simulink model "Bebop2_sim_only_vis_faster_real_cubic_working_backup"  (R2018a)
settings: Solver=VariableStepAuto  StartTime=0.0  StopTime=25  FixedStep=.04  MaxStep=1.00  MinStep=0.005  RelTol=1e-6  AbsTol=1e-6
values from neighbouring files (symbols this model uses):
  flightplan = [dist,0,height,deg2rad(090) ... (first row only)    [compare_cubic_spline_1.m]    (also in initialize_race_realtime.m; initialize_race_realtime_backup_cubic.m; plot_sim.m = [ 4.348, -0.278, height, deg2rad(  0); test_b_spline.m)
  FOV = 1.05    [initialize_race_realtime.m]    (also in initialize_race_realtime_backup_cubic.m)
  g = 9.81    [initialize_race_no_realtime.m]    (also in initialize_race_realtime.m; initialize_race_realtime_backup_cubic.m; moving_average_rls_own.m = P(i-1)*meas*(lambda+meas*P(i-1)*meas)^-1)
  gate_size = 1.4    [initialize_race_realtime.m]    (also in initialize_race_realtime_backup_cubic.m)
  gates = sim_gates(:,:,1)    [eval_sim.m]    (also in initialize_race_realtime.m = [dist,0,height,deg2rad(110); initialize_race_realtime_backup_cubic.m = [dist,0,height,deg2rad(110); plot_sim.m)
  I = [1 0 0 ... (first row only)    [Bebop_sim_init.m]    (also in initialize_race_no_realtime.m; initialize_race_realtime.m; initialize_race_realtime_backup_cubic.m; moving_averge_rls_download.m = ones(1,N))
  init_std_dev = [1.0*ones(1,3),deg2rad(30)]    [initialize_race_realtime.m]    (also in initialize_race_realtime_backup_cubic.m)
  Initial_ori = [0 0 pi/4]    [initialize_race_no_realtime.m]    (also in initialize_race_realtime.m; initialize_race_realtime_backup_cubic.m)
  Initial_pos = [0 0 1]    [Bebop_sim_init.m]    (also in initialize_race_no_realtime.m = [0 -3 2]; initialize_race_realtime.m = [0 -3 2]; initialize_race_realtime_backup_cubic.m = [0 -3 2])
  Initial_vel_e = max_vel*[1,0,0]    [initialize_race_realtime.m]    (also in initialize_race_realtime_backup_cubic.m)
  m = 0.68    [calc_plot_spline.m]    (also in calc_spline.m; compare_cubic_spline_1.m = vpasolve(e,r); compare_cubic_spline_2.m = r/3*(-sin(dp)+sqrt(sin(dp)^2-6*cos(dp)+6)); initialize_race_no_realtime.m = 2)
  max_rot_Z = (90)*pi/180    (= 1.57079632679)    [Bebop_sim_init.m]    (also in initialize_race_no_realtime.m = 1.0471975512; initialize_race_realtime.m; initialize_race_realtime_backup_cubic.m; run_batch1.m = list_agility(idx_agility)*max_rot_Z)
  max_theta_X = (40)*pi/180    (= 0.698131700798)    [Bebop_sim_init.m]    (also in initialize_race_no_realtime.m = 0.13962634016; initialize_race_realtime.m = 1.308996939; initialize_race_realtime_backup_cubic.m = 1.308996939; run_batch1.m = list_agility(idx_agility)*max_theta_X)
  max_theta_Y = (40)*pi/180    (= 0.698131700798)    [Bebop_sim_init.m]    (also in initialize_race_no_realtime.m = 0.13962634016; initialize_race_realtime.m = 1.308996939; initialize_race_realtime_backup_cubic.m = 1.308996939; run_batch1.m = list_agility(idx_agility)*max_theta_Y)
  max_v_Z = .5    (= 0.5)    [Bebop_sim_init.m]    (also in initialize_race_no_realtime.m = 1; initialize_race_realtime.m = 3; initialize_race_realtime_backup_cubic.m = 3; run_batch1.m = list_agility(idx_agility)*max_v_Z)
  max_vel = 1.5    [initialize_race_realtime.m]    (also in initialize_race_realtime_backup_cubic.m; run_batch1.m = list_speed(idx_speed); run_batch2.m = list_speed(idx_speed); run_batch3.m = list_speed(idx_speed))
undefined symbols (not defined in the file or in its folder): fspecial, gray, Rec, SDTV
libraries: simulink x11, sharedtransform x11, visiontextngfix x4, visiontransforms x3, aerolibactuator x2, aerolibutil x2, vrlib x2, visionanalysis x2, visionconversions x2, shared6dof x1, visionstatistics x1, visionsinks x1
(part 2 of 4)

== system Bebop2_sim_only_vis_faster_real_cubic_working_backup/Vision System/Harris Corners ==
  Threshold : Inport
  Corner Detection : visionanalysis/Corner Detection  method=Harris corner detection (Harris & Stephens)  factor=0.01  filter=fspecial('gaussian', [1 9], 3)  thrInten=0.1  thrAngle=157.5  output=Obsolete9b  outputInUse=Corner location  maxNum=5  thrMetric=0.01  neighborSize=[25 25]  isOutVarDim=on  accumMode=Binary point scaling  accumWordLength=32  accumFracLength=0  prodOutputMode=Binary point scaling  prodOutputWordLength=32  prodOutputFracLength=0  memoryMode=Binary point scaling  memoryWordLength=32  memoryFracLength=0  firstCoeffMode=Specify word length  firstCoeffWordLength=16  firstCoeffFracLength=17  roundingMode=Floor  overflowMode=off
      settings: SourceProductName=Computer Vision System Toolbox  SourceProductBaseCode=VP
  Gaussian Pyramid : visiontransforms/Gaussian Pyramid  Commented=on  operation=Expand  level=1  source=Specify via dialog  a=0.375  coef=fspecial('gaussian', [1 9], 3)  hiddenCoef=fspecial('gaussian', [1 9], 3)  firstCoeffMode=Specify word length  firstCoeffWordLength=16  firstCoeffFracLength=17  outputMode=Binary point scaling  outputWordLength=32  outputFracLength=10  prodOutputMode=Binary point scaling  prodOutputWordLength=32  prodOutputFracLength=10  roundingMode=Floor  overflowMode=off
      settings: SourceProductName=Computer Vision System Toolbox  SourceProductBaseCode=VP
  Video Viewer2 : VideoViewer  Commented=on  colormapValue=gray(256)  FigPos=[76 898 768 763]
  Corners : Outport
  wires:
  Threshold/1 -> Gaussian Pyramid/1, Corner Detection/1
  Gaussian Pyramid/1 -> Video Viewer2/1
  Corner Detection/1 -> Corners/1

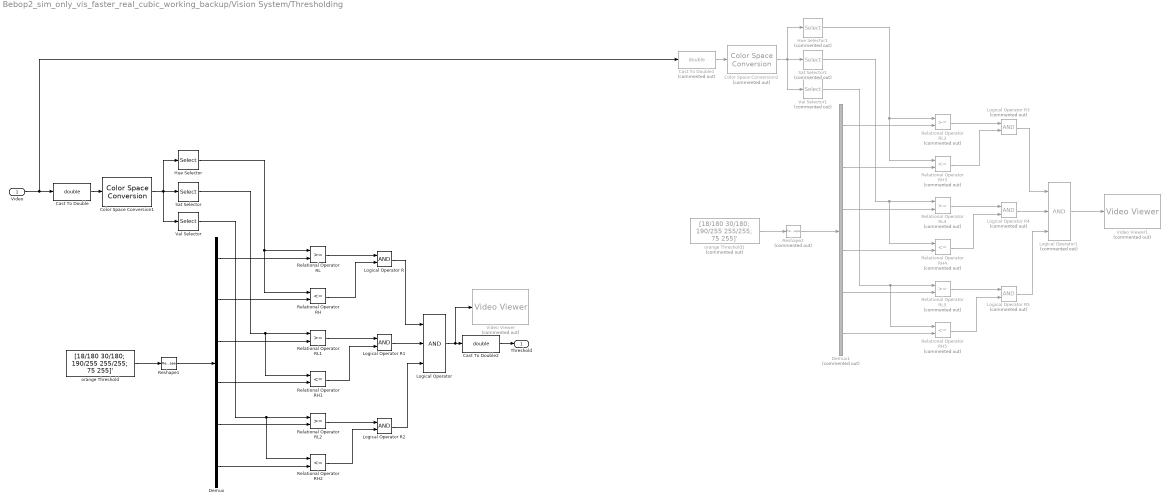
== system Bebop2_sim_only_vis_faster_real_cubic_working_backup/Vision System/Thresholding ==
  "Video " : Inport
  Cast To Double : DataTypeConversion  OutDataTypeStr=double
  Cast To Double1 : DataTypeConversion  Commented=on  OutDataTypeStr=double
  Cast To Double2 : DataTypeConversion  OutDataTypeStr=double
  Color Space Conversion1 : visionconversions/Color Space  Conversion  conversion=Obsolete  conversionActive=R'G'B' to HSV  wp_str=D65  rec=Rec. 601 (SDTV)  sys=1125/60/2:1  imagePorts=One multidimensional signal
      settings: SourceProductName=Computer Vision System Toolbox
  Color Space Conversion2 : visionconversions/Color Space  Conversion  Commented=on  conversion=Obsolete  conversionActive=R'G'B' to HSV  wp_str=D65  rec=Rec. 601 (SDTV)  sys=1125/60/2:1  imagePorts=One multidimensional signal
      settings: SourceProductName=Computer Vision System Toolbox
  Demux : Demux  Outputs=6
  Demux1 : Demux  Commented=on  Outputs=6
  Hue Selector : Selector  NumberOfDimensions=3  IndexMode=Zero-based  InputPortWidth=3  IndexOptions=Select all,Select all,Index vector (dialog)  Indices=[1 3],1,0  OutputSizes=1,1,1
  Hue Selector1 : Selector  Commented=on  NumberOfDimensions=3  InputPortWidth=3  IndexOptions=Select all,Select all,Index vector (dialog)  Indices=[1 3],1,1  OutputSizes=1,1,1
  Logical Operator : Logic  Inputs=3  AllPortsSameDT=off  OutDataTypeStr=boolean
  Logical Operator R : Logic  AllPortsSameDT=off  OutDataTypeStr=boolean
  Logical Operator R1 : Logic  AllPortsSameDT=off  OutDataTypeStr=boolean
  Logical Operator R2 : Logic  AllPortsSameDT=off  OutDataTypeStr=boolean
  Logical Operator R3 : Logic  Commented=on  AllPortsSameDT=off  OutDataTypeStr=boolean
  Logical Operator R4 : Logic  Commented=on  AllPortsSameDT=off  OutDataTypeStr=boolean
  Logical Operator R5 : Logic  Commented=on  AllPortsSameDT=off  OutDataTypeStr=boolean
  Logical Operator1 : Logic  Commented=on  Inputs=3  AllPortsSameDT=off  OutDataTypeStr=boolean
  Relational Operator RH : RelationalOperator  Operator=<=  OutDataTypeStr=boolean  RndMeth=Nearest
  Relational Operator RH1 : RelationalOperator  Operator=<=  OutDataTypeStr=boolean  RndMeth=Nearest
  Relational Operator RH2 : RelationalOperator  Operator=<=  OutDataTypeStr=boolean  RndMeth=Nearest
  Relational Operator RH3 : RelationalOperator  Commented=on  Operator=<=  OutDataTypeStr=boolean  RndMeth=Nearest
  Relational Operator RH4 : RelationalOperator  Commented=on  Operator=<=  OutDataTypeStr=boolean  RndMeth=Nearest
  Relational Operator RH5 : RelationalOperator  Commented=on  Operator=<=  OutDataTypeStr=boolean  RndMeth=Nearest
  Relational Operator RL : RelationalOperator  OutDataTypeStr=boolean  RndMeth=Nearest
  Relational Operator RL1 : RelationalOperator  OutDataTypeStr=boolean  RndMeth=Nearest
  Relational Operator RL2 : RelationalOperator  OutDataTypeStr=boolean  RndMeth=Nearest
  Relational Operator RL3 : RelationalOperator  Commented=on  OutDataTypeStr=boolean  RndMeth=Nearest
  Relational Operator RL4 : RelationalOperator  Commented=on  OutDataTypeStr=boolean  RndMeth=Nearest
  Relational Operator RL5 : RelationalOperator  Commented=on  OutDataTypeStr=boolean  RndMeth=Nearest
  Reshape1 : Reshape
  Reshape2 : Reshape  Commented=on
  Sat Selector : Selector  NumberOfDimensions=3  IndexMode=Zero-based  InputPortWidth=3  IndexOptions=Select all,Select all,Index vector (dialog)  Indices=[1 3],1,1  OutputSizes=1,1,1
  Sat Selector1 : Selector  Commented=on  NumberOfDimensions=3  InputPortWidth=3  IndexOptions=Select all,Select all,Index vector (dialog)  Indices=[1 3],1,2  OutputSizes=1,1,1
  Val Selector : Selector  NumberOfDimensions=3  IndexMode=Zero-based  InputPortWidth=3  IndexOptions=Select all,Select all,Index vector (dialog)  Indices=[1 3],1,2  OutputSizes=1,1,1
  Val Selector1 : Selector  Commented=on  NumberOfDimensions=3  InputPortWidth=3  IndexOptions=Select all,Select all,Index vector (dialog)  Indices=[1 3],1,3  OutputSizes=1,1,1
  Video Viewer : VideoViewer  Commented=on  colormapValue=gray(256)  FigPos=[833 898 768 793]
  Video Viewer1 : VideoViewer  Commented=on  colormapValue=gray(256)  FigPos=[823 898 778 793]
  orange Threshold : Constant  Value=[18/180 30/180; 190/255 255/255; 75 255]'  OutDataTypeStr=double
  orange Threshold1 : Constant  Commented=on  Value=[18/180 30/180; 190/255 255/255; 75 255]'  OutDataTypeStr=double
  Threshold : Outport
  wires:
  Color Space Conversion1/1 -> Val Selector/1, Sat Selector/1, Hue Selector/1
  Demux/6 -> Relational Operator RH2/2
  Val Selector/1 -> Relational Operator RH2/1, Relational Operator RL2/1
  Demux/3 -> Relational Operator RL1/2
  Relational Operator RL/1 -> Logical Operator R/1
  Demux/2 -> Relational Operator RH/2
  orange Threshold/1 -> Reshape1/1
  Cast To Double/1 -> Color Space Conversion1/1
  Demux/5 -> Relational Operator RL2/2
  Hue Selector/1 -> Relational Operator RH/1, Relational Operator RL/1
  Logical Operator R/1 -> Logical Operator/1
  Relational Operator RH/1 -> Logical Operator R/2
  Demux/1 -> Relational Operator RL/2
  Demux/4 -> Relational Operator RH1/2
  Reshape1/1 -> Demux/1
  Logical Operator R1/1 -> Logical Operator/2
  Relational Operator RH1/1 -> Logical Operator R1/2
  Sat Selector/1 -> Relational Operator RH1/1, Relational Operator RL1/1
  Relational Operator RL1/1 -> Logical Operator R1/1
  Relational Operator RH2/1 -> Logical Operator R2/2
  Relational Operator RL2/1 -> Logical Operator R2/1
  Logical Operator R2/1 -> Logical Operator/3
  Logical Operator/1 -> Video Viewer/1, Cast To Double2/1
  Demux1/5 -> Relational Operator RL5/2
  Relational Operator RH3/1 -> Logical Operator R3/2
  orange Threshold1/1 -> Reshape2/1
  Demux1/1 -> Relational Operator RL3/2
  Relational Operator RH4/1 -> Logical Operator R4/2
  Demux1/4 -> Relational Operator RH4/2
  Relational Operator RH5/1 -> Logical Operator R5/2
  Logical Operator R5/1 -> Logical Operator1/3
  Relational Operator RL4/1 -> Logical Operator R4/1
  Demux1/6 -> Relational Operator RH5/2
  Demux1/2 -> Relational Operator RH3/2
  Reshape2/1 -> Demux1/1
  Logical Operator1/1 -> Video Viewer1/1
  Hue Selector1/1 -> Relational Operator RH3/1, Relational Operator RL3/1
  Color Space Conversion2/1 -> Val Selector1/1, Sat Selector1/1, Hue Selector1/1
  Logical Operator R3/1 -> Logical Operator1/1
  Cast To Double1/1 -> Color Space Conversion2/1
  Demux1/3 -> Relational Operator RL4/2
  Relational Operator RL3/1 -> Logical Operator R3/1
  Val Selector1/1 -> Relational Operator RH5/1, Relational Operator RL5/1
  Relational Operator RL5/1 -> Logical Operator R5/1
  Logical Operator R4/1 -> Logical Operator1/2
  "Video "/1 -> Cast To Double1/1, Cast To Double/1
  Sat Selector1/1 -> Relational Operator RH4/1, Relational Operator RL4/1
  Cast To Double2/1 -> Threshold/1

== system Bebop2_sim_only_vis_faster_real_cubic_working_backup/Vision System/calculate corners ==
  In1 : Inport
  Action Port : ActionPort  PropagateVarSize=During execution  ActionType=then
  calculate corners : MATLAB Function  TreatAsAtomicUnit=on
  Out1 : Outport
  wires:
  In1/1 -> calculate corners/1(corners)
  calculate corners/1(corners_four) -> Out1/1

== system Bebop2_sim_only_vis_faster_real_cubic_working_backup/conv/global2strange drone ==
  note: rotm2axang(m1*m2)
  note: eul2rotm([-pi/2, 0, pi/2])
  note: eul2rotm([euler(3),euler(2),euler(1)])
  euler global : Inport
  Constant : Constant  Value=pi/2
  Constant1 : Constant  Value=0
  Direction Cosine Matrix to Quaternions : sharedtransform/Direction Cosine Matrix  to Quaternions  aMode=0  action=None  tolerance=eps(2)
      settings: SourceProductName=Aerospace Blockset  SourceProductBaseCode=AE
  Gain : Gain  Gain=-1
  Gain2 : Gain  Gain=-1
  Gain3 : Gain  Gain=[-1,-1,-1,1]
  MATLAB Function : MATLAB Function  Commented=on  TreatAsAtomicUnit=on
  MATLAB Function1 : MATLAB Function  TreatAsAtomicUnit=on
  Matrix Multiply : Product  Multiplication=Matrix(*)
  Rotation Angles to Direction Cosine Matrix : sharedtransform/Rotation Angles to Direction Cosine Matrix  rotationOrder=XYZ  aMode=aMode
      settings: SourceProductBaseCode=AE
  Rotation Angles to Direction Cosine Matrix1 : sharedtransform/Rotation Angles to Direction Cosine Matrix  rotationOrder=XYZ  aMode=aMode
      settings: SourceProductBaseCode=AE
  Vector Concatenate : Concatenate  NumInputs=3
  axang strange : Outport
  wires:
  Constant/1 -> Vector Concatenate/3, Gain/1
  Constant1/1 -> Vector Concatenate/2
  Gain/1 -> Vector Concatenate/1
  Rotation Angles to Direction Cosine Matrix/1 -> Matrix Multiply/2
  euler global/1 -> Gain2/1
  Rotation Angles to Direction Cosine Matrix1/1 -> Matrix Multiply/1
  Matrix Multiply/1 -> Direction Cosine Matrix to Quaternions/1
  MATLAB Function1/1(axang) -> Gain3/1
  Vector Concatenate/1 -> Rotation Angles to Direction Cosine Matrix/1
  Gain2/1 -> Rotation Angles to Direction Cosine Matrix1/1
  Direction Cosine Matrix to Quaternions/1 -> MATLAB Function1/1(q)
  Gain3/1 -> axang strange/1

== system Bebop2_sim_only_vis_faster_real_cubic_working_backup/Control/Control algorithm/Create Path Frame ==
  Velocity Vector : Inport
  Invert 3x3 Matrix : aerolibutil/Invert  3x3 Matrix
  Make X Vector : Subsystem
  Make Y Vector : Subsystem
  Make Z Vector : Subsystem
  Matrix Concatenate : Concatenate  NumInputs=3  Mode=Multidimensional array  ConcatenateDimension=2
  Rotation Matrix : Outport
  wires:
  Velocity Vector/1 -> Make Z Vector/1(Velocity Vector), Make X Vector/1(Velocity Vector), Make Y Vector/1(Velocity Vector)
  Make Y Vector/1(Y Vector) -> Matrix Concatenate/2
  Make X Vector/1(X Vector) -> Matrix Concatenate/1
  Make Z Vector/1(Z Vector) -> Matrix Concatenate/3
  Matrix Concatenate/1 -> Invert 3x3 Matrix/1
  Invert 3x3 Matrix/1 -> Rotation Matrix/1

== system Bebop2_sim_only_vis_faster_real_cubic_working_backup/Control/Control algorithm/Hdg Controller R ==
  delta yaw : Inport
  Atan2 : Trigonometry  Operator=atan2
  Cos : Trigonometry  Operator=sincos
  PID Controller 0.075 : simulink/Continuous/PID Controller  Controller=PID  TimeDomain=Continuous-time  SampleTime=-1  IntegratorMethod=Forward Euler  FilterMethod=Forward Euler  Form=Parallel  UseFilter=on  ControllerParametersSource=internal  P=9  I=0  D=.9  N=100  InitialConditionSource=internal  InitialConditionForIntegrator=0  InitialConditionForFilter=0  ExternalReset=none  LimitOutput=off  UpperSaturationLimit=inf  LowerSaturationLimit=-inf  LinearizeAsGain=on  AntiWindupMode=none  Kb=1  TrackingMode=off  Kt=1  PParamMin=[]  PParamMax=[]  IParamMin=[]  IParamMax=[]  DParamMin=[]  DParamMax=[]  NParamMin=[]  NParamMax=[]  KbParamMin=[]  KbParamMax=[]  KtParamMin=[]  KtParamMax=[]  POutMin=[]  POutMax=[]  IOutMin=[]  IOutMax=[]  DOutMin=[]  DOutMax=[]  NOutMin=[]  NOutMax=[]  KbOutMin=[]  KbOutMax=[]  KtOutMin=[]  KtOutMax=[]  IntegratorOutMin=[]  IntegratorOutMax=[]  FilterOutMin=[]  FilterOutMax=[]  SumOutMin=[]  SumOutMax=[]  SumI1OutMin=[]  SumI1OutMax=[]  SumI2OutMin=[]  SumI2OutMax=[]  SumI3OutMin=[]  SumI3OutMax=[]  SumDOutMin=[]  SumDOutMax=[]  SaturationOutMin=[]  SaturationOutMax=[]  IntegratorContinuousStateAttributes=''  IntegratorStateMustResolveToSignalObject=off  IntegratorRTWStateStorageClass=Auto  FilterContinuousStateAttributes=''  FilterStateMustResolveToSignalObject=off  FilterRTWStateStorageClass=Auto  DifferentiatorICPrevScaledInput=0  DifferentiatorOutMin=[]  DifferentiatorOutMax=[]  FilterDiffOutCoefMin=[]  FilterDiffOutCoefMax=[]  SumDenOutMin=[]  SumDenOutMax=[]  SumNumOutMin=[]  SumNumOutMax=[]  ReciprocalOutMin=[]  ReciprocalOutMax=[]  DivideOutMin=[]  DivideOutMax=[]  TunerSelectOption=Transfer Function Based (PID Tuner App)
  PID Controller 0.15 : simulink/Continuous/PID Controller  Controller=PID  TimeDomain=Continuous-time  SampleTime=-1  IntegratorMethod=Forward Euler  FilterMethod=Forward Euler  Form=Parallel  UseFilter=on  ControllerParametersSource=internal  P=4  I=0  D=0  N=100  InitialConditionSource=internal  InitialConditionForIntegrator=0  InitialConditionForFilter=0  ExternalReset=none  LimitOutput=off  UpperSaturationLimit=inf  LowerSaturationLimit=-inf  LinearizeAsGain=on  AntiWindupMode=none  Kb=1  TrackingMode=off  Kt=1  PParamMin=[]  PParamMax=[]  IParamMin=[]  IParamMax=[]  DParamMin=[]  DParamMax=[]  NParamMin=[]  NParamMax=[]  KbParamMin=[]  KbParamMax=[]  KtParamMin=[]  KtParamMax=[]  POutMin=[]  POutMax=[]  IOutMin=[]  IOutMax=[]  DOutMin=[]  DOutMax=[]  NOutMin=[]  NOutMax=[]  KbOutMin=[]  KbOutMax=[]  KtOutMin=[]  KtOutMax=[]  IntegratorOutMin=[]  IntegratorOutMax=[]  FilterOutMin=[]  FilterOutMax=[]  SumOutMin=[]  SumOutMax=[]  SumI1OutMin=[]  SumI1OutMax=[]  SumI2OutMin=[]  SumI2OutMax=[]  SumI3OutMin=[]  SumI3OutMax=[]  SumDOutMin=[]  SumDOutMax=[]  SaturationOutMin=[]  SaturationOutMax=[]  IntegratorContinuousStateAttributes=''  IntegratorStateMustResolveToSignalObject=off  IntegratorRTWStateStorageClass=Auto  FilterContinuousStateAttributes=''  FilterStateMustResolveToSignalObject=off  FilterRTWStateStorageClass=Auto  DifferentiatorICPrevScaledInput=0  DifferentiatorOutMin=[]  DifferentiatorOutMax=[]  FilterDiffOutCoefMin=[]  FilterDiffOutCoefMax=[]  SumDenOutMin=[]  SumDenOutMax=[]  SumNumOutMin=[]  SumNumOutMax=[]  ReciprocalOutMin=[]  ReciprocalOutMax=[]  DivideOutMin=[]  DivideOutMax=[]  TunerSelectOption=Transfer Function Based (PID Tuner App)
  PID Controller 0.15 p : simulink/Continuous/PID Controller  Controller=PID  TimeDomain=Continuous-time  SampleTime=-1  IntegratorMethod=Forward Euler  FilterMethod=Forward Euler  Form=Parallel  UseFilter=on  ControllerParametersSource=internal  P=3  I=0  D=0  N=100  InitialConditionSource=internal  InitialConditionForIntegrator=0  InitialConditionForFilter=0  ExternalReset=none  LimitOutput=off  UpperSaturationLimit=inf  LowerSaturationLimit=-inf  LinearizeAsGain=on  AntiWindupMode=none  Kb=1  TrackingMode=off  Kt=1  PParamMin=[]  PParamMax=[]  IParamMin=[]  IParamMax=[]  DParamMin=[]  DParamMax=[]  NParamMin=[]  NParamMax=[]  KbParamMin=[]  KbParamMax=[]  KtParamMin=[]  KtParamMax=[]  POutMin=[]  POutMax=[]  IOutMin=[]  IOutMax=[]  DOutMin=[]  DOutMax=[]  NOutMin=[]  NOutMax=[]  KbOutMin=[]  KbOutMax=[]  KtOutMin=[]  KtOutMax=[]  IntegratorOutMin=[]  IntegratorOutMax=[]  FilterOutMin=[]  FilterOutMax=[]  SumOutMin=[]  SumOutMax=[]  SumI1OutMin=[]  SumI1OutMax=[]  SumI2OutMin=[]  SumI2OutMax=[]  SumI3OutMin=[]  SumI3OutMax=[]  SumDOutMin=[]  SumDOutMax=[]  SaturationOutMin=[]  SaturationOutMax=[]  IntegratorContinuousStateAttributes=''  IntegratorStateMustResolveToSignalObject=off  IntegratorRTWStateStorageClass=Auto  FilterContinuousStateAttributes=''  FilterStateMustResolveToSignalObject=off  FilterRTWStateStorageClass=Auto  DifferentiatorICPrevScaledInput=0  DifferentiatorOutMin=[]  DifferentiatorOutMax=[]  FilterDiffOutCoefMin=[]  FilterDiffOutCoefMax=[]  SumDenOutMin=[]  SumDenOutMax=[]  SumNumOutMin=[]  SumNumOutMax=[]  ReciprocalOutMin=[]  ReciprocalOutMax=[]  DivideOutMin=[]  DivideOutMax=[]  TunerSelectOption=Transfer Function Based (PID Tuner App)
  yaw rate : Outport
  wires:
  delta yaw/1 -> Cos/1  "delta yaw"
  Cos/1 -> Atan2/1
  PID Controller 0.075/1 -> yaw rate/1  "yaw rate"
  Atan2/1 -> PID Controller 0.075/1  "d yaw"
  Cos/2 -> Atan2/2

== system Bebop2_sim_only_vis_faster_real_cubic_working_backup/Control/Control algorithm/Orientation to 3D yaw rotation ==
  Drone yaw : Inport
  Constant1 : Constant  Value=0
  Rotation Angles to Direction Cosine Matrix : sharedtransform/Rotation Angles to Direction Cosine Matrix  rotationOrder=ZYX  aMode=aMode
      settings: SourceProductBaseCode=AE
  Vector Concatenate : Concatenate  NumInputs=3
  rot matrix : Outport
  wires:
  Constant1/1 -> Vector Concatenate/2, Vector Concatenate/3
  Vector Concatenate/1 -> Rotation Angles to Direction Cosine Matrix/1
  Drone yaw/1 -> Vector Concatenate/1  "yaw"
  Rotation Angles to Direction Cosine Matrix/1 -> rot matrix/1  "rot matrix"

== system Bebop2_sim_only_vis_faster_real_cubic_working_backup/Control/Control algorithm/Vel Controller X,Y1 ==
  note: 0.075
  note: 0.15
  note: 0.075
  delta V traj : Inport
  Demux1 : Demux  Outputs=3
  Gain3 : Gain  Gain=2
  Gain4 : Gain  Gain=8
  Gain5 : Gain  Gain=2.5
  Gain6 : Gain  Gain=.75
  Gain7 : Gain  Gain=3
  Gain8 : Gain  Gain=1.25
  Mux : Mux  Inputs=3
  PID Controller1 : simulink/Continuous/PID Controller  Controller=PID  TimeDomain=Continuous-time  SampleTime=-1  IntegratorMethod=Forward Euler  FilterMethod=Forward Euler  Form=Parallel  UseFilter=on  ControllerParametersSource=internal  P=2  I=0  D=0  N=100  InitialConditionSource=internal  InitialConditionForIntegrator=0  InitialConditionForFilter=0  ExternalReset=none  LimitOutput=off  UpperSaturationLimit=inf  LowerSaturationLimit=-inf  LinearizeAsGain=on  AntiWindupMode=none  Kb=1  TrackingMode=off  Kt=1  PParamMin=[]  PParamMax=[]  IParamMin=[]  IParamMax=[]  DParamMin=[]  DParamMax=[]  NParamMin=[]  NParamMax=[]  KbParamMin=[]  KbParamMax=[]  KtParamMin=[]  KtParamMax=[]  POutMin=[]  POutMax=[]  IOutMin=[]  IOutMax=[]  DOutMin=[]  DOutMax=[]  NOutMin=[]  NOutMax=[]  KbOutMin=[]  KbOutMax=[]  KtOutMin=[]  KtOutMax=[]  IntegratorOutMin=[]  IntegratorOutMax=[]  FilterOutMin=[]  FilterOutMax=[]  SumOutMin=[]  SumOutMax=[]  SumI1OutMin=[]  SumI1OutMax=[]  SumI2OutMin=[]  SumI2OutMax=[]  SumI3OutMin=[]  SumI3OutMax=[]  SumDOutMin=[]  SumDOutMax=[]  SaturationOutMin=[]  SaturationOutMax=[]  IntegratorContinuousStateAttributes=''  IntegratorStateMustResolveToSignalObject=off  IntegratorRTWStateStorageClass=Auto  FilterContinuousStateAttributes=''  FilterStateMustResolveToSignalObject=off  FilterRTWStateStorageClass=Auto  DifferentiatorICPrevScaledInput=0  DifferentiatorOutMin=[]  DifferentiatorOutMax=[]  FilterDiffOutCoefMin=[]  FilterDiffOutCoefMax=[]  SumDenOutMin=[]  SumDenOutMax=[]  SumNumOutMin=[]  SumNumOutMax=[]  ReciprocalOutMin=[]  ReciprocalOutMax=[]  DivideOutMin=[]  DivideOutMax=[]  TunerSelectOption=Transfer Function Based (PID Tuner App)
  PID Controller2 : simulink/Continuous/PID Controller  Controller=PID  TimeDomain=Continuous-time  SampleTime=-1  IntegratorMethod=Forward Euler  FilterMethod=Forward Euler  Form=Parallel  UseFilter=on  ControllerParametersSource=internal  P=6  I=0  D=.9  N=100  InitialConditionSource=internal  InitialConditionForIntegrator=0  InitialConditionForFilter=0  ExternalReset=none  LimitOutput=off  UpperSaturationLimit=inf  LowerSaturationLimit=-inf  LinearizeAsGain=on  AntiWindupMode=none  Kb=1  TrackingMode=off  Kt=1  PParamMin=[]  PParamMax=[]  IParamMin=[]  IParamMax=[]  DParamMin=[]  DParamMax=[]  NParamMin=[]  NParamMax=[]  KbParamMin=[]  KbParamMax=[]  KtParamMin=[]  KtParamMax=[]  POutMin=[]  POutMax=[]  IOutMin=[]  IOutMax=[]  DOutMin=[]  DOutMax=[]  NOutMin=[]  NOutMax=[]  KbOutMin=[]  KbOutMax=[]  KtOutMin=[]  KtOutMax=[]  IntegratorOutMin=[]  IntegratorOutMax=[]  FilterOutMin=[]  FilterOutMax=[]  SumOutMin=[]  SumOutMax=[]  SumI1OutMin=[]  SumI1OutMax=[]  SumI2OutMin=[]  SumI2OutMax=[]  SumI3OutMin=[]  SumI3OutMax=[]  SumDOutMin=[]  SumDOutMax=[]  SaturationOutMin=[]  SaturationOutMax=[]  IntegratorContinuousStateAttributes=''  IntegratorStateMustResolveToSignalObject=off  IntegratorRTWStateStorageClass=Auto  FilterContinuousStateAttributes=''  FilterStateMustResolveToSignalObject=off  FilterRTWStateStorageClass=Auto  DifferentiatorICPrevScaledInput=0  DifferentiatorOutMin=[]  DifferentiatorOutMax=[]  FilterDiffOutCoefMin=[]  FilterDiffOutCoefMax=[]  SumDenOutMin=[]  SumDenOutMax=[]  SumNumOutMin=[]  SumNumOutMax=[]  ReciprocalOutMin=[]  ReciprocalOutMax=[]  DivideOutMin=[]  DivideOutMax=[]  TunerSelectOption=Transfer Function Based (PID Tuner App)
  PID Controller3 : simulink/Continuous/PID Controller  Controller=PID  TimeDomain=Continuous-time  SampleTime=-1  IntegratorMethod=Forward Euler  FilterMethod=Forward Euler  Form=Parallel  UseFilter=on  ControllerParametersSource=internal  P=1  I=0  D=0  N=100  InitialConditionSource=internal  InitialConditionForIntegrator=0  InitialConditionForFilter=0  ExternalReset=none  LimitOutput=off  UpperSaturationLimit=inf  LowerSaturationLimit=-inf  LinearizeAsGain=on  AntiWindupMode=none  Kb=1  TrackingMode=off  Kt=1  PParamMin=[]  PParamMax=[]  IParamMin=[]  IParamMax=[]  DParamMin=[]  DParamMax=[]  NParamMin=[]  NParamMax=[]  KbParamMin=[]  KbParamMax=[]  KtParamMin=[]  KtParamMax=[]  POutMin=[]  POutMax=[]  IOutMin=[]  IOutMax=[]  DOutMin=[]  DOutMax=[]  NOutMin=[]  NOutMax=[]  KbOutMin=[]  KbOutMax=[]  KtOutMin=[]  KtOutMax=[]  IntegratorOutMin=[]  IntegratorOutMax=[]  FilterOutMin=[]  FilterOutMax=[]  SumOutMin=[]  SumOutMax=[]  SumI1OutMin=[]  SumI1OutMax=[]  SumI2OutMin=[]  SumI2OutMax=[]  SumI3OutMin=[]  SumI3OutMax=[]  SumDOutMin=[]  SumDOutMax=[]  SaturationOutMin=[]  SaturationOutMax=[]  IntegratorContinuousStateAttributes=''  IntegratorStateMustResolveToSignalObject=off  IntegratorRTWStateStorageClass=Auto  FilterContinuousStateAttributes=''  FilterStateMustResolveToSignalObject=off  FilterRTWStateStorageClass=Auto  DifferentiatorICPrevScaledInput=0  DifferentiatorOutMin=[]  DifferentiatorOutMax=[]  FilterDiffOutCoefMin=[]  FilterDiffOutCoefMax=[]  SumDenOutMin=[]  SumDenOutMax=[]  SumNumOutMin=[]  SumNumOutMax=[]  ReciprocalOutMin=[]  ReciprocalOutMax=[]  DivideOutMin=[]  DivideOutMax=[]  TunerSelectOption=Transfer Function Based (PID Tuner App)
  PID Controller4 : simulink/Continuous/PID Controller  Controller=PID  TimeDomain=Continuous-time  SampleTime=-1  IntegratorMethod=Forward Euler  FilterMethod=Forward Euler  Form=Parallel  UseFilter=on  ControllerParametersSource=internal  P=5  I=0  D=.4  N=100  InitialConditionSource=internal  InitialConditionForIntegrator=0  InitialConditionForFilter=0  ExternalReset=none  LimitOutput=off  UpperSaturationLimit=inf  LowerSaturationLimit=-inf  LinearizeAsGain=on  AntiWindupMode=none  Kb=1  TrackingMode=off  Kt=1  PParamMin=[]  PParamMax=[]  IParamMin=[]  IParamMax=[]  DParamMin=[]  DParamMax=[]  NParamMin=[]  NParamMax=[]  KbParamMin=[]  KbParamMax=[]  KtParamMin=[]  KtParamMax=[]  POutMin=[]  POutMax=[]  IOutMin=[]  IOutMax=[]  DOutMin=[]  DOutMax=[]  NOutMin=[]  NOutMax=[]  KbOutMin=[]  KbOutMax=[]  KtOutMin=[]  KtOutMax=[]  IntegratorOutMin=[]  IntegratorOutMax=[]  FilterOutMin=[]  FilterOutMax=[]  SumOutMin=[]  SumOutMax=[]  SumI1OutMin=[]  SumI1OutMax=[]  SumI2OutMin=[]  SumI2OutMax=[]  SumI3OutMin=[]  SumI3OutMax=[]  SumDOutMin=[]  SumDOutMax=[]  SaturationOutMin=[]  SaturationOutMax=[]  IntegratorContinuousStateAttributes=''  IntegratorStateMustResolveToSignalObject=off  IntegratorRTWStateStorageClass=Auto  FilterContinuousStateAttributes=''  FilterStateMustResolveToSignalObject=off  FilterRTWStateStorageClass=Auto  DifferentiatorICPrevScaledInput=0  DifferentiatorOutMin=[]  DifferentiatorOutMax=[]  FilterDiffOutCoefMin=[]  FilterDiffOutCoefMax=[]  SumDenOutMin=[]  SumDenOutMax=[]  SumNumOutMin=[]  SumNumOutMax=[]  ReciprocalOutMin=[]  ReciprocalOutMax=[]  DivideOutMin=[]  DivideOutMax=[]  TunerSelectOption=Transfer Function Based (PID Tuner App)
  PID Controller5 : simulink/Continuous/PID Controller  Controller=PID  TimeDomain=Continuous-time  SampleTime=-1  IntegratorMethod=Forward Euler  FilterMethod=Forward Euler  Form=Parallel  UseFilter=on  ControllerParametersSource=internal  P=3  I=0  D=0  N=100  InitialConditionSource=internal  InitialConditionForIntegrator=0  InitialConditionForFilter=0  ExternalReset=none  LimitOutput=off  UpperSaturationLimit=inf  LowerSaturationLimit=-inf  LinearizeAsGain=on  AntiWindupMode=none  Kb=1  TrackingMode=off  Kt=1  PParamMin=[]  PParamMax=[]  IParamMin=[]  IParamMax=[]  DParamMin=[]  DParamMax=[]  NParamMin=[]  NParamMax=[]  KbParamMin=[]  KbParamMax=[]  KtParamMin=[]  KtParamMax=[]  POutMin=[]  POutMax=[]  IOutMin=[]  IOutMax=[]  DOutMin=[]  DOutMax=[]  NOutMin=[]  NOutMax=[]  KbOutMin=[]  KbOutMax=[]  KtOutMin=[]  KtOutMax=[]  IntegratorOutMin=[]  IntegratorOutMax=[]  FilterOutMin=[]  FilterOutMax=[]  SumOutMin=[]  SumOutMax=[]  SumI1OutMin=[]  SumI1OutMax=[]  SumI2OutMin=[]  SumI2OutMax=[]  SumI3OutMin=[]  SumI3OutMax=[]  SumDOutMin=[]  SumDOutMax=[]  SaturationOutMin=[]  SaturationOutMax=[]  IntegratorContinuousStateAttributes=''  IntegratorStateMustResolveToSignalObject=off  IntegratorRTWStateStorageClass=Auto  FilterContinuousStateAttributes=''  FilterStateMustResolveToSignalObject=off  FilterRTWStateStorageClass=Auto  DifferentiatorICPrevScaledInput=0  DifferentiatorOutMin=[]  DifferentiatorOutMax=[]  FilterDiffOutCoefMin=[]  FilterDiffOutCoefMax=[]  SumDenOutMin=[]  SumDenOutMax=[]  SumNumOutMin=[]  SumNumOutMax=[]  ReciprocalOutMin=[]  ReciprocalOutMax=[]  DivideOutMin=[]  DivideOutMax=[]  TunerSelectOption=Transfer Function Based (PID Tuner App)
  PID Controller6 : simulink/Continuous/PID Controller  Controller=PID  TimeDomain=Continuous-time  SampleTime=-1  IntegratorMethod=Forward Euler  FilterMethod=Forward Euler  Form=Parallel  UseFilter=on  ControllerParametersSource=internal  P=1  I=0  D=0  N=100  InitialConditionSource=internal  InitialConditionForIntegrator=0  InitialConditionForFilter=0  ExternalReset=none  LimitOutput=off  UpperSaturationLimit=inf  LowerSaturationLimit=-inf  LinearizeAsGain=on  AntiWindupMode=none  Kb=1  TrackingMode=off  Kt=1  PParamMin=[]  PParamMax=[]  IParamMin=[]  IParamMax=[]  DParamMin=[]  DParamMax=[]  NParamMin=[]  NParamMax=[]  KbParamMin=[]  KbParamMax=[]  KtParamMin=[]  KtParamMax=[]  POutMin=[]  POutMax=[]  IOutMin=[]  IOutMax=[]  DOutMin=[]  DOutMax=[]  NOutMin=[]  NOutMax=[]  KbOutMin=[]  KbOutMax=[]  KtOutMin=[]  KtOutMax=[]  IntegratorOutMin=[]  IntegratorOutMax=[]  FilterOutMin=[]  FilterOutMax=[]  SumOutMin=[]  SumOutMax=[]  SumI1OutMin=[]  SumI1OutMax=[]  SumI2OutMin=[]  SumI2OutMax=[]  SumI3OutMin=[]  SumI3OutMax=[]  SumDOutMin=[]  SumDOutMax=[]  SaturationOutMin=[]  SaturationOutMax=[]  IntegratorContinuousStateAttributes=''  IntegratorStateMustResolveToSignalObject=off  IntegratorRTWStateStorageClass=Auto  FilterContinuousStateAttributes=''  FilterStateMustResolveToSignalObject=off  FilterRTWStateStorageClass=Auto  DifferentiatorICPrevScaledInput=0  DifferentiatorOutMin=[]  DifferentiatorOutMax=[]  FilterDiffOutCoefMin=[]  FilterDiffOutCoefMax=[]  SumDenOutMin=[]  SumDenOutMax=[]  SumNumOutMin=[]  SumNumOutMax=[]  ReciprocalOutMin=[]  ReciprocalOutMax=[]  DivideOutMin=[]  DivideOutMax=[]  TunerSelectOption=Transfer Function Based (PID Tuner App)
  accel traj : Outport
  wires:
  delta V traj/1 -> Demux1/1  "delta V traj"
  Demux1/2 -> PID Controller2/1
  Demux1/1 -> PID Controller4/1
  Demux1/3 -> PID Controller3/1
  PID Controller3/1 -> Mux/3
  PID Controller4/1 -> Mux/1
  Mux/1 -> accel traj/1  "accel traj"
  PID Controller2/1 -> Mux/2

== system Bebop2_sim_only_vis_faster_real_cubic_working_backup/Gate info/Yaw2Axang1/Subsystem ==
  note: u(2)/sqrt(1-u(1)*u(1)), u(3)/sqrt(1-u(1)*u(1)), u(4)/sqrt(1-u(1)*u(1)),
  In1 : Inport
  Fcn : Fcn  Expr=2*acos(u(1))
  Fcn1 : Fcn  Expr=u(2)/sqrt(1-u(1)*u(1))
  Fcn2 : Fcn  Expr=u(3)/sqrt(1-u(1)*u(1))
  Fcn3 : Fcn  Expr=u(4)/sqrt(1-u(1)*u(1))
  Vector Concatenate : Concatenate  NumInputs=4
  Out1 : Outport
  wires:
  In1/1 -> Fcn/1, Fcn3/1, Fcn2/1, Fcn1/1
  Fcn1/1 -> Vector Concatenate/1
  Fcn2/1 -> Vector Concatenate/2
  Fcn3/1 -> Vector Concatenate/3
  Fcn/1 -> Vector Concatenate/4
  Vector Concatenate/1 -> Out1/1

== system Bebop2_sim_only_vis_faster_real_cubic_working_backup/Gate info/Yaw2Axang2/Subsystem ==
  note: u(2)/sqrt(1-u(1)*u(1)), u(3)/sqrt(1-u(1)*u(1)), u(4)/sqrt(1-u(1)*u(1)),
  In1 : Inport
  Fcn : Fcn  Expr=2*acos(u(1))
  Fcn1 : Fcn  Expr=u(2)/sqrt(1-u(1)*u(1))
  Fcn2 : Fcn  Expr=u(3)/sqrt(1-u(1)*u(1))
  Fcn3 : Fcn  Expr=u(4)/sqrt(1-u(1)*u(1))
  Vector Concatenate : Concatenate  NumInputs=4
  Out1 : Outport
  wires:
  In1/1 -> Fcn/1, Fcn3/1, Fcn2/1, Fcn1/1
  Fcn1/1 -> Vector Concatenate/1
  Fcn2/1 -> Vector Concatenate/2
  Fcn3/1 -> Vector Concatenate/3
  Fcn/1 -> Vector Concatenate/4
  Vector Concatenate/1 -> Out1/1

== system Bebop2_sim_only_vis_faster_real_cubic_working_backup/Gate info/Yaw2Axang5/Subsystem ==
  note: u(2)/sqrt(1-u(1)*u(1)), u(3)/sqrt(1-u(1)*u(1)), u(4)/sqrt(1-u(1)*u(1)),
  In1 : Inport
  Fcn : Fcn  Expr=2*acos(u(1))
  Fcn1 : Fcn  Expr=u(2)/sqrt(1-u(1)*u(1))
  Fcn2 : Fcn  Expr=u(3)/sqrt(1-u(1)*u(1))
  Fcn3 : Fcn  Expr=u(4)/sqrt(1-u(1)*u(1))
  Vector Concatenate : Concatenate  NumInputs=4
  Out1 : Outport
  wires:
  In1/1 -> Fcn/1, Fcn3/1, Fcn2/1, Fcn1/1
  Fcn1/1 -> Vector Concatenate/1
  Fcn2/1 -> Vector Concatenate/2
  Fcn3/1 -> Vector Concatenate/3
  Fcn/1 -> Vector Concatenate/4
  Vector Concatenate/1 -> Out1/1

== system Bebop2_sim_only_vis_faster_real_cubic_working_backup/Gate info/Yaw2Axang6/Subsystem ==
  note: u(2)/sqrt(1-u(1)*u(1)), u(3)/sqrt(1-u(1)*u(1)), u(4)/sqrt(1-u(1)*u(1)),
  In1 : Inport
  Fcn : Fcn  Expr=2*acos(u(1))
  Fcn1 : Fcn  Expr=u(2)/sqrt(1-u(1)*u(1))
  Fcn2 : Fcn  Expr=u(3)/sqrt(1-u(1)*u(1))
  Fcn3 : Fcn  Expr=u(4)/sqrt(1-u(1)*u(1))
  Vector Concatenate : Concatenate  NumInputs=4
  Out1 : Outport
  wires:
  In1/1 -> Fcn/1, Fcn3/1, Fcn2/1, Fcn1/1
  Fcn1/1 -> Vector Concatenate/1
  Fcn2/1 -> Vector Concatenate/2
  Fcn3/1 -> Vector Concatenate/3
  Fcn/1 -> Vector Concatenate/4
  Vector Concatenate/1 -> Out1/1

== system Bebop2_sim_only_vis_faster_real_cubic_working_backup/Navigation/calculate desired/If Action Subsystem ==
  In1 : Inport
  Action Port : ActionPort  ActionType=then
  Out1 : Outport
  wires:
  In1/1 -> Out1/1

== system Bebop2_sim_only_vis_faster_real_cubic_working_backup/Navigation/calculate desired/If Action Subsystem1 ==
  In1 : Inport
  Action Port : ActionPort  ActionType=else
  Out1 : Outport
  wires:
  In1/1 -> Out1/1

== system Bebop2_sim_only_vis_faster_real_cubic_working_backup/Navigation/calculate desired/calc pos B(d) ==
  note: B(d) = (1-d).^3*P0 + 3*(1-d).^2.*d*P1 + 3*(1-d).*d.^2*P2 + d.^3*P3;
  P0 : Inport
  P1 : Inport  Port=2
  P2 : Inport  Port=3
  P3 : Inport  Port=4
  d : Inport  Port=5
  Add3 : Sum  Inputs=++++
  Constant1 : Constant
  Constant2 : Constant  Value=3
  Constant3 : Constant  Value=3
  Gain : Gain  Gain=3
  Gain1 : Gain  Gain=3
  Multiply : Product
  Multiply1 : Product  Inputs=3
  Multiply8 : Product  Inputs=3
  Multiply9 : Product
  Power : Math  Operator=square  SaturateOnIntegerOverflow=on
  Power1 : Math  Operator=pow  SaturateOnIntegerOverflow=on
  Power2 : Math  Operator=square  SaturateOnIntegerOverflow=on
  Power3 : Math  Operator=pow  SaturateOnIntegerOverflow=on
  Sum1 : Sum  Inputs=|+-
  "old, quadratic" : Subsystem  Commented=on
  pos : Outport
  wires:
  Gain/1 -> Add3/2
  Gain1/1 -> Add3/3
  P1/1 -> Multiply1/1
  P0/1 -> Multiply/1
  P2/1 -> Multiply8/1
  P3/1 -> Multiply9/1
  Multiply/1 -> Add3/1
  Multiply1/1 -> Gain/1
  Multiply8/1 -> Gain1/1
  Multiply9/1 -> Add3/4
  Add3/1 -> pos/1
  Constant1/1 -> Sum1/1
  d/1 -> Sum1/2, Multiply1/3, Power2/1, Power3/1  "d"
  Power/1 -> Multiply1/2
  Power1/1 -> Multiply/2
  Power2/1 -> Multiply8/3
  Power3/1 -> Multiply9/2
  Constant2/1 -> Power1/2
  Constant3/1 -> Power3/2
  Sum1/1 -> Multiply8/2, Power/1, Power1/1

== system Bebop2_sim_only_vis_faster_real_cubic_working_backup/Navigation/calculate desired/calculate direction B'(d) ==
  note: B'(d) = 3(1-d)^2(P1-P0) + 6*(1-d)*d*(P2-P1) + 3d^2(P3-P2)
  P0 : Inport
  P1 : Inport  Port=2
  P2 : Inport  Port=3
  P3 : Inport  Port=4
  d : Inport  Port=5
  vel : Inport  Port=6
  Add3 : Sum  Inputs=+++
  Constant3 : Constant
  Gain : Gain  Gain=6
  Gain1 : Gain  Gain=3
  Gain2 : Gain  Gain=3
  Make Unit : Subsystem
  Minus : Sum  Inputs=-+
  Minus1 : Sum  Inputs=-+
  Minus2 : Sum  Inputs=-+
  Multiply : Product
  Multiply1 : Product  Inputs=3
  Multiply2 : Product
  Multiply8 : Product
  Power1 : Math  Operator=square  SaturateOnIntegerOverflow=on
  Power2 : Math  Operator=square  SaturateOnIntegerOverflow=on
  Sum1 : Sum  Inputs=|+-
  "old, quadratic" : Subsystem  Commented=on
  global vel des : Outport
  wires:
  Sum1/1 -> Multiply1/2, Power1/1
  Minus1/1 -> Multiply1/1
  Minus/1 -> Multiply/1
  Gain/1 -> Add3/2
  Gain1/1 -> Add3/3
  Multiply1/1 -> Gain/1
  Minus2/1 -> Multiply8/1
  Constant3/1 -> Sum1/1
  Multiply/1 -> Gain2/1
  Multiply8/1 -> Gain1/1
  Power2/1 -> Multiply8/2
  Power1/1 -> Multiply/2
  d/1 -> Sum1/2, Power2/1, Multiply1/3  "d"
  Gain2/1 -> Add3/1
  P0/1 -> Minus/1  "P0"
  P1/1 -> Minus/2, Minus1/1  "P1"
  P2/1 -> Minus1/2, Minus2/1  "P2"
  P3/1 -> Minus2/2  "P3"
  Multiply2/1 -> global vel des/1
  Add3/1 -> Make Unit/1(Vector)
  Make Unit/1(Unit Vector) -> Multiply2/1
  vel/1 -> Multiply2/2  "vel"

== system Bebop2_sim_only_vis_faster_real_cubic_working_backup/Navigation/calculate desired/min gate distance ==
  Constant2 : Constant  Value=gate_size
  Constant3 : Constant  Value=FOV
  Divide : Product  Inputs=*/
  Gain1 : Gain  Gain=0.5
  Gain2 : Gain  Gain=0.5
  Tan : Trigonometry  Operator=tan
  min gate dist : Outport
  wires:
  Constant3/1 -> Gain2/1
  Constant2/1 -> Gain1/1
  Gain1/1 -> Divide/1
  Gain2/1 -> Tan/1
  Divide/1 -> min gate dist/1  "min dist"
  Tan/1 -> Divide/2

== system Bebop2_sim_only_vis_faster_real_cubic_working_backup/Navigation/calculate velocity/Create Path Frame ==
  Velocity Vector : Inport
  Invert 3x3 Matrix : aerolibutil/Invert  3x3 Matrix
  Make X Vector : Subsystem
  Make Y Vector : Subsystem
  Make Z Vector : Subsystem
  Matrix Concatenate : Concatenate  NumInputs=3  Mode=Multidimensional array  ConcatenateDimension=2
  Rotation Matrix : Outport
  wires:
  Velocity Vector/1 -> Make Z Vector/1(Velocity Vector), Make X Vector/1(Velocity Vector), Make Y Vector/1(Velocity Vector)
  Make Y Vector/1(Y Vector) -> Matrix Concatenate/2
  Make X Vector/1(X Vector) -> Matrix Concatenate/1
  Make Z Vector/1(Z Vector) -> Matrix Concatenate/3
  Matrix Concatenate/1 -> Invert 3x3 Matrix/1
  Invert 3x3 Matrix/1 -> Rotation Matrix/1

== system Bebop2_sim_only_vis_faster_real_cubic_working_backup/Navigation/calculate velocity/Exp offset ==
  note: y=s-(s-b) e^{-k(x-d)}
  distance : Inport
  Exp : Math  SaturateOnIntegerOverflow=on
  Gain : Gain  Gain=-1
  Minus : Sum  Inputs=-+
  Multiply : Product
  Multiply1 : Product
  Sum : Sum  Inputs=-+|
  Sum1 : Sum  Inputs=|-+
  b : Constant  Value=.5
  d : Constant  Value=4
  k : Constant  Value=-1
  s : Constant  Value=.2
  max offset : Outport
  wires:
  distance/1 -> Sum/2
  d/1 -> Sum/1
  k/1 -> Gain/1
  Gain/1 -> Multiply/2
  Sum/1 -> Multiply/1
  Multiply/1 -> Exp/1
  b/1 -> Sum1/1
  Exp/1 -> Multiply1/1
  Sum1/1 -> Multiply1/2
  s/1 -> Minus/2, Sum1/2
  Multiply1/1 -> Minus/1
  Minus/1 -> max offset/1

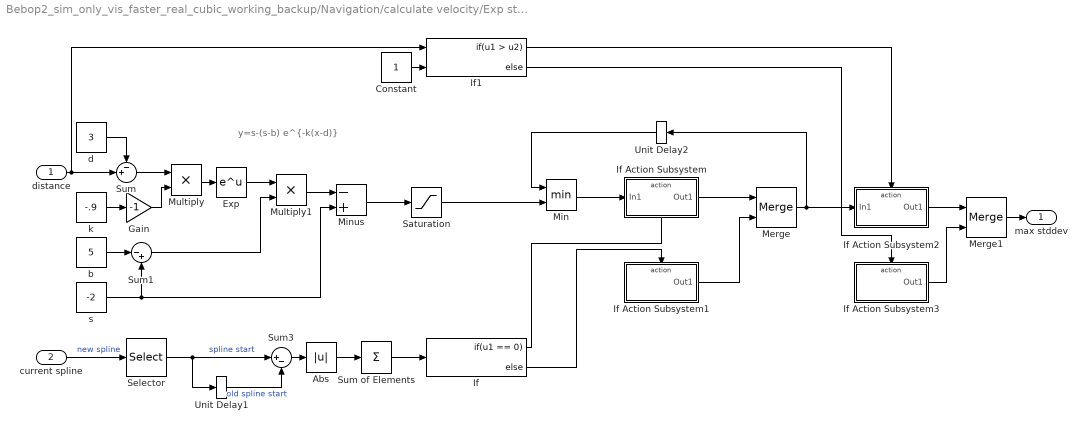
== system Bebop2_sim_only_vis_faster_real_cubic_working_backup/Navigation/calculate velocity/Exp std.dev ==
  note: y=s-(s-b) e^{-k(x-d)}
  distance : Inport
  current spline : Inport  Port=2
  Abs : Abs
  Constant : Constant
  Exp : Math  SaturateOnIntegerOverflow=on
  Gain : Gain  Gain=-1
  If : If  IfExpression=u1 == 0
  If Action Subsystem : Subsystem  TreatAsAtomicUnit=on
  If Action Subsystem1 : Subsystem  TreatAsAtomicUnit=on
  If Action Subsystem2 : Subsystem  TreatAsAtomicUnit=on
  If Action Subsystem3 : Subsystem  TreatAsAtomicUnit=on
  If1 : If  NumInputs=2  IfExpression=u1 > u2
  Merge : Merge
  Merge1 : Merge
  Min : MinMax  Inputs=2
  Minus : Sum  Inputs=-+
  Multiply : Product
  Multiply1 : Product
  Saturation : Saturate  UpperLimit=99  LowerLimit=0.5
  Selector : Selector  NumberOfDimensions=2  IndexMode=Zero-based  InputPortWidth=3  IndexOptions=Index vector (dialog),Select all  Indices=0,[0 1 2]  OutputSizes=1,1
  Sum : Sum  Inputs=-+|
  Sum of Elements : Sum  Inputs=+
  Sum1 : Sum  Inputs=|-+
  Sum3 : Sum  Inputs=|+-
  Unit Delay1 : UnitDelay  SampleTime=-1
  Unit Delay2 : UnitDelay  InitialCondition=20  SampleTime=-1
  b : Constant  Value=5
  d : Constant  Value=3
  k : Constant  Value=-.9
  s : Constant  Value=-2
  max stddev : Outport
  wires:
  Sum1/1 -> Multiply1/2
  k/1 -> Gain/1
  distance/1 -> If1/1, Sum/2
  Sum/1 -> Multiply/1
  Exp/1 -> Multiply1/1
  Multiply1/1 -> Minus/1
  d/1 -> Sum/1
  b/1 -> Sum1/1
  Multiply/1 -> Exp/1
  Minus/1 -> Saturation/1
  Gain/1 -> Multiply/2
  s/1 -> Minus/2, Sum1/2
  Saturation/1 -> Min/2
  If/2 -> If Action Subsystem1/Action
  If Action Subsystem/1(Out1) -> Merge/1
  current spline/1 -> Selector/1  "new spline"
  Sum3/1 -> Abs/1
  If/1 -> If Action Subsystem/Action
  If Action Subsystem1/1(Out1) -> Merge/2
  Sum of Elements/1 -> If/1
  Unit Delay1/1 -> Sum3/2  "old spline start"
  Selector/1 -> Unit Delay1/1, Sum3/1  "spline start"
  Abs/1 -> Sum of Elements/1
  Min/1 -> If Action Subsystem/1(In1)
  Unit Delay2/1 -> Min/1
  Merge/1 -> If Action Subsystem2/1(In1), Unit Delay2/1
  Constant/1 -> If1/2
  If1/1 -> If Action Subsystem2/Action
  If1/2 -> If Action Subsystem3/Action
  Merge1/1 -> max stddev/1
  If Action Subsystem2/1(Out1) -> Merge1/1
  If Action Subsystem3/1(Out1) -> Merge1/2

== system Bebop2_sim_only_vis_faster_real_cubic_working_backup/Navigation/calculate velocity/If Action Subsystem ==
  In1 : Inport
  Action Port : ActionPort  ActionType=then
  Saturation3 : Saturate  UpperLimit=1  LowerLimit=0
  Out1 : Outport
  wires:
  In1/1 -> Saturation3/1
  Saturation3/1 -> Out1/1

== system Bebop2_sim_only_vis_faster_real_cubic_working_backup/Navigation/calculate velocity/If Action Subsystem1 ==
  In1 : Inport
  Action Port : ActionPort  ActionType=else
  Out1 : Outport
  wires:
  In1/1 -> Out1/1

== system Bebop2_sim_only_vis_faster_real_cubic_working_backup/Navigation/calculate velocity/calculate direction B'(d) ==
  note: B'(d) = 3(1-d)^2(P1-P0) + 6*(1-d)*d*(P2-P1) + 3d^2(P3-P2)
  spline : Inport
  d : Inport  Port=2
  Add3 : Sum  Inputs=+++
  Constant3 : Constant
  Gain : Gain  Gain=6
  Gain1 : Gain  Gain=3
  Gain2 : Gain  Gain=3
  Minus : Sum  Inputs=-+
  Minus1 : Sum  Inputs=-+
  Minus2 : Sum  Inputs=-+
  Multiply : Product
  Multiply1 : Product  Inputs=3
  Multiply8 : Product
  Power1 : Math  Operator=square  SaturateOnIntegerOverflow=on
  Power2 : Math  Operator=square  SaturateOnIntegerOverflow=on
  Selector1 : Selector  NumberOfDimensions=2  IndexMode=Zero-based  InputPortWidth=3  IndexOptions=Index vector (dialog),Select all  Indices=0,[0 1 2]  OutputSizes=1,1
  Selector2 : Selector  NumberOfDimensions=2  IndexMode=Zero-based  InputPortWidth=3  IndexOptions=Index vector (dialog),Select all  Indices=1,[0 1 2]  OutputSizes=1,1
  Selector3 : Selector  NumberOfDimensions=2  IndexMode=Zero-based  InputPortWidth=3  IndexOptions=Index vector (dialog),Select all  Indices=2,[0 1 2]  OutputSizes=1,1
  Selector4 : Selector  NumberOfDimensions=2  IndexMode=Zero-based  InputPortWidth=3  IndexOptions=Index vector (dialog),Select all  Indices=3,[0 1 2]  OutputSizes=1,1
  Sum1 : Sum  Inputs=|+-
  "old, quadratic" : Subsystem  Commented=on
  direction : Outport
  wires:
  Sum1/1 -> Multiply1/2, Power1/1
  Minus1/1 -> Multiply1/1
  Minus/1 -> Multiply/1
  Gain/1 -> Add3/2
  Gain1/1 -> Add3/3
  Multiply1/1 -> Gain/1
  Minus2/1 -> Multiply8/1
  Constant3/1 -> Sum1/1
  Multiply/1 -> Gain2/1
  Multiply8/1 -> Gain1/1
  Power2/1 -> Multiply8/2
  Power1/1 -> Multiply/2
  d/1 -> Sum1/2, Power2/1, Multiply1/3  "d"
  Gain2/1 -> Add3/1
  Add3/1 -> direction/1
  Selector1/1 -> Minus/1  "P0"
  Selector3/1 -> Minus2/1, Minus1/2  "P2"
  spline/1 -> Selector2/1, Selector1/1, Selector4/1, Selector3/1  "spline para"
  Selector2/1 -> Minus1/1, Minus/2  "P1"
  Selector4/1 -> Minus2/2  "P3"

== system Bebop2_sim_only_vis_faster_real_cubic_working_backup/Navigation/calculate velocity/min spd ==
  In1 : Inport
  Abs : Abs
  Add : Sum  Inputs=+-
  Constant : Constant  Value=0.01
  Constant1 : Constant  Value=0.5
  Minus : Sum  Inputs=+-
  Multiply : Product
  Saturation : Saturate  UpperLimit=0  LowerLimit=-1
  Scope : Scope  NumInputPorts=7
  Sign : Signum
  Sign1 : Signum
  Sum : Sum  Inputs=|++
  Out1 : Outport
  wires:
  In1/1 -> Scope/1, Add/1, Sign/1, Abs/1
  Abs/1 -> Minus/1
  Constant/1 -> Minus/2
  Minus/1 -> Scope/4, Saturation/1
  Saturation/1 -> Scope/5, Multiply/1
  Sum/1 -> Sign1/1
  Multiply/1 -> Scope/2, Add/2
  Add/1 -> Scope/3, Out1/1
  Constant1/1 -> Sum/2
  Sign1/1 -> Multiply/2
  Sign/1 -> Sum/1

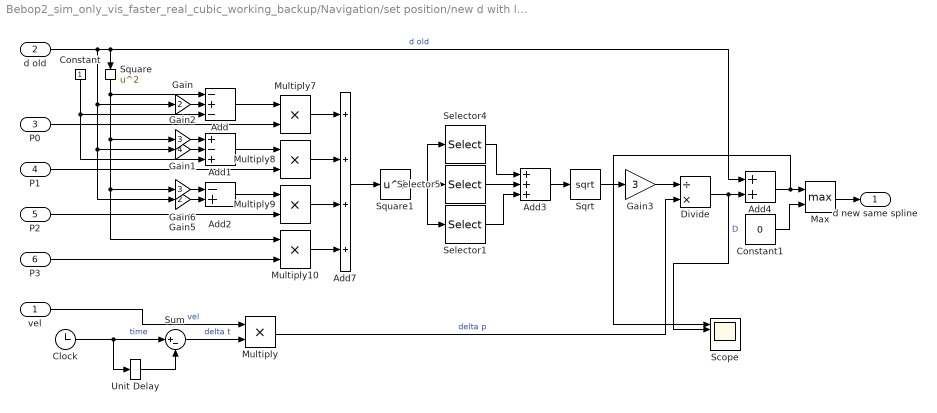
== system Bebop2_sim_only_vis_faster_real_cubic_working_backup/Navigation/set position/new d with linearization ==
  vel : Inport
  d old : Inport  Port=2
  P0 : Inport  Port=3
  P1 : Inport  Port=4
  P2 : Inport  Port=5
  P3 : Inport  Port=6
  Add : Sum  Inputs=-+-
  Add1 : Sum  Inputs=+-+
  Add2 : Sum  Inputs=-+
  Add3 : Sum  Inputs=+++
  Add4 : Sum
  Add7 : Sum  Inputs=++++
  Clock : Clock
  Constant : Constant
  Constant1 : Constant  Value=0
  Divide : Product  Inputs=/*
  Gain : Gain  Gain=2
  Gain1 : Gain  Gain=4
  Gain2 : Gain  Gain=3
  Gain3 : Gain  Gain=3
  Gain5 : Gain  Gain=2
  Gain6 : Gain  Gain=3
  Max : MinMax  Function=max  Inputs=2
  Multiply{,7..10} (5 alike) : Product
  Scope : Scope  NumInputPorts=5
  Selector1 : Selector  IndexMode=Zero-based  InputPortWidth=3  IndexOptions=Index vector (dialog)  Indices=2  OutputSizes=1
  Selector4 : Selector  IndexMode=Zero-based  InputPortWidth=3  IndexOptions=Index vector (dialog)  Indices=0  OutputSizes=1
  Selector5 : Selector  IndexMode=Zero-based  InputPortWidth=3  IndexOptions=Index vector (dialog)  Indices=1  OutputSizes=1
  Sqrt : Sqrt  SaturateOnIntegerOverflow=on
  Square : Math  Operator=square  SaturateOnIntegerOverflow=on
  Square1 : Math  Operator=square  SaturateOnIntegerOverflow=on
  Sum : Sum  Inputs=|+-
  Unit Delay : UnitDelay  SampleTime=-1
  d new same spline : Outport
  wires:
  Add7/1 -> Square1/1
  Multiply8/1 -> Add7/2
  Multiply9/1 -> Add7/3
  Square/1 -> Multiply10/1, Gain6/1, Gain2/1, Add/1
  Gain/1 -> Add/2
  Constant/1 -> Add1/3, Add/3
  Gain2/1 -> Add1/1
  Gain1/1 -> Add1/2
  Gain6/1 -> Add2/1
  Gain5/1 -> Add2/2
  Multiply10/1 -> Add7/4
  Add2/1 -> Multiply9/1
  Add1/1 -> Multiply8/1
  Add/1 -> Multiply7/1
  P0/1 -> Multiply7/2
  P1/1 -> Multiply8/2
  P2/1 -> Multiply9/2
  P3/1 -> Multiply10/2
  Multiply7/1 -> Add7/1
  Selector5/1 -> Add3/2
  d old/1 -> Add4/1, Square/1, Gain/1, Gain5/1, Gain1/1  "d old"
  Multiply/1 -> Divide/2  "delta p"
  Gain3/1 -> Divide/1
  Divide/1 -> Scope/2, Add4/2  "D"
  Selector4/1 -> Add3/1
  Add3/1 -> Sqrt/1
  Square1/1 -> Selector1/1, Selector4/1, Selector5/1
  Sqrt/1 -> Gain3/1
  Selector1/1 -> Add3/3
  Sum/1 -> Multiply/2  "delta t"
  Unit Delay/1 -> Sum/2
  vel/1 -> Multiply/1  "vel"
  Clock/1 -> Unit Delay/1, Sum/1  "time"
  Add4/1 -> Max/1, Scope/1
  Constant1/1 -> Max/2
  Max/1 -> d new same spline/1
